simulink model "DSB_SC_AM_System"  (R2024a)
settings: Solver=VariableStepAuto  StartTime=0.0  StopTime=10.0  RelTol=1e-3
libraries: dspfdesign x2, commchan3 x1
settings Model: Creator=alice  LastModifiedBy=alice

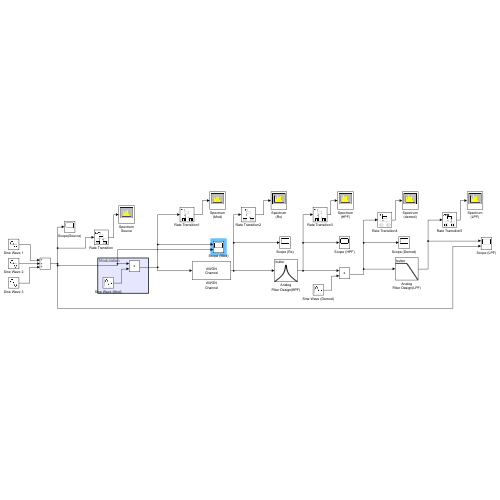
[thumbnail: Simulink's stored preview of the top-level diagram]
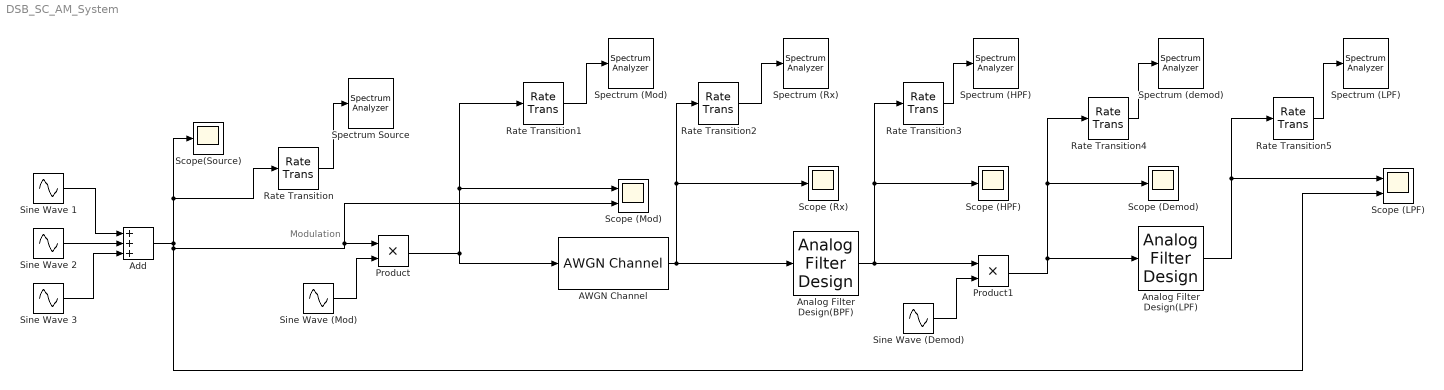
== system DSB_SC_AM_System ==
  note: Modulation
  AWGN Channel : commchan3/AWGN Channel  LegacyMode=off  NoiseMethod=Variance  noiseMode="Signal to noise ratio  (SNR)"  EbNo=10  EsNo=10  SNR=10  BitsPerSymbol=1  SignalPower=1  SamplesPerSymbol=1  SymbolPeriod=1  VarianceSource=Parameter  Variance=1e-2  RandomStream=mt19937ar with seed  Seed=67  SimulateUsing=Code generation
  Add : Sum  Inputs=+++
  Analog Filter Design(BPF) : dspfdesign/Analog Filter Design  method=Butterworth  filttype=Bandpass  N=8  Wlo=14300*2*pi  Whi=15800*2*pi  Rp=2  Rs=40
  Analog Filter Design(LPF) : dspfdesign/Analog Filter Design  method=Butterworth  filttype=Lowpass  N=8  Wlo=800*2*pi  Whi=80  Rp=2  Rs=40
  Product : Product
  Product1 : Product
  Rate Transition{,1..5} (6 alike) : RateTransition  OutPortSampleTime=2e-5
  Scope (Demod) : Scope
  Scope (HPF) : Scope
  Scope (LPF) : Scope  NumInputPorts=2
  Scope (Mod) : Scope  NumInputPorts=2
  Scope (Rx) : Scope
  Scope(Source) : Scope
  Sine Wave (Demod) : Sin  Frequency=30000*pi  Phase=pi/2  SampleTime=0
  Sine Wave (Mod) : Sin  Frequency=30000*pi  Phase=pi/2  SampleTime=0
  Sine Wave 1 : Sin  Frequency=1000*pi  SampleTime=0
  Sine Wave 2 : Sin  Amplitude=3  Frequency=600*pi  SampleTime=0
  Sine Wave 3 : Sin  Amplitude=1.5  Frequency=1200*pi  SampleTime=0
  Spectrum (HPF) : SpectrumAnalyzer  WindowPosition=[240.000000,150.000000,800.000000,500.000000,]  ScopeFrameLocation=window  YLimits=[-94.70638307,41.05528627]
  Spectrum (LPF) : SpectrumAnalyzer  WindowPosition=[240.000000,150.000000,800.000000,500.000000,]  ScopeFrameLocation=window  YLimits=[-251.44956334,58.15554882]
  Spectrum (Mod) : SpectrumAnalyzer  WindowPosition=[1.000000,49.000000,1280.000000,729.000000,]  ScopeFrameLocation=window  RBW=5  YLimits=[-243.51897953,57.61458242]  SelectedToolstripTab=spectrumAnalyzerToolstrip.channelMeasurementsTab
  Spectrum (Rx) : SpectrumAnalyzer  WindowPosition=[1.000000,49.000000,1280.000000,729.000000,]  ScopeFrameLocation=window  YLimits=[-30.14187097,33.88966257]  SelectedToolstripTab=spectrumAnalyzerToolstrip.estimationTab
  Spectrum (demod) : SpectrumAnalyzer  WindowPosition=[240.000000,150.000000,800.000000,500.000000,]  ScopeFrameLocation=window  YLimits=[-98.06362305,41.11115053]
  Spectrum Source : SpectrumAnalyzer  WindowPosition=[266.000000,185.000000,800.000000,500.000000,]  ScopeFrameLocation=window  YLimits=[-246.51481572,64.63688443]  SelectedToolstripTab=spectrumAnalyzerToolstrip.channelMeasurementsTab
  wires:
  Sine Wave 1/1 -> Add/1
  Sine Wave 2/1 -> Add/2
  Sine Wave 3/1 -> Add/3
  Add/1 -> Scope (LPF)/2, Scope (Mod)/2, Product/1, Rate Transition/1, Scope(Source)/1
  Sine Wave (Mod)/1 -> Product/2
  Rate Transition/1 -> Spectrum Source/1
  Product/1 -> AWGN Channel/1, Scope (Mod)/1, Rate Transition1/1
  Rate Transition1/1 -> Spectrum (Mod)/1
  Rate Transition2/1 -> Spectrum (Rx)/1
  AWGN Channel/1 -> Rate Transition2/1, Scope (Rx)/1, Analog Filter Design(BPF)/1
  Analog Filter Design(BPF)/1 -> Product1/1, Scope (HPF)/1, Rate Transition3/1
  Rate Transition3/1 -> Spectrum (HPF)/1
  Sine Wave (Demod)/1 -> Product1/2
  Rate Transition4/1 -> Spectrum (demod)/1
  Product1/1 -> Analog Filter Design(LPF)/1, Scope (Demod)/1, Rate Transition4/1
  Rate Transition5/1 -> Spectrum (LPF)/1
  Analog Filter Design(LPF)/1 -> Scope (LPF)/1, Rate Transition5/1
